simulink model "traffic_moore_stateflow"  (R2020b)
settings: Solver=VariableStepAuto  StartTime=0.0  StopTime=10.0  RelTol=1e-3
settings Model: Creator=ADMIN  LastModifiedBy=ADMIN

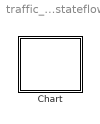
== system traffic_moore_stateflow ==
  Chart : Stateflow chart  TreatAsAtomicUnit=on

== stateflow chart traffic_moore_stateflow/Chart ==
  settings: stateMachineType=MOORE_MACHINE
